simulink model "MotorControl"  (R2016a)
settings: Solver=VariableStepAuto  StartTime=0.0  StopTime=2  MaxStep=.01  RelTol=1e-3
libraries: simulink x3
settings Model: Creator=Dillon  LastModifiedBy=Dillon

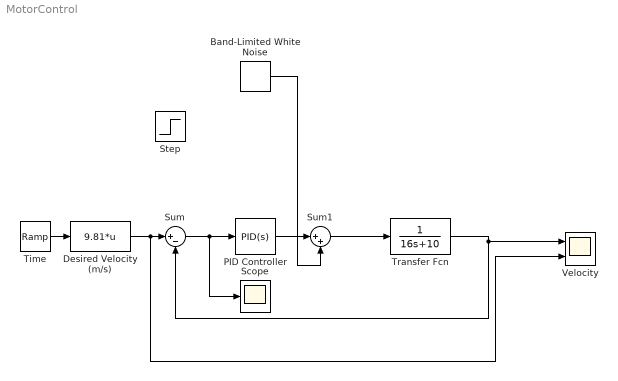
== system MotorControl ==
  Band-Limited White Noise : simulink/Sources/Band-Limited White Noise  Cov=[100]  Ts=0.1  seed=[23341]
  Desired Velocity (m/s) : Fcn  Expr=9.81*u
  PID Controller : simulink/Continuous/PID Controller  Controller=PID  TimeDomain=Continuous-time  SampleTime=-1  IntegratorMethod=Forward Euler  FilterMethod=Forward Euler  Form=Parallel  UseFilter=on  ControllerParametersSource=internal  P=100  I=1000  D=10  N=100  InitialConditionSource=internal  InitialConditionForIntegrator=0  InitialConditionForFilter=0  ExternalReset=none  LimitOutput=off  UpperSaturationLimit=inf  LowerSaturationLimit=-inf  LinearizeAsGain=on  AntiWindupMode=none  Kb=1  TrackingMode=off  Kt=1  PParamMin=[]  PParamMax=[]  IParamMin=[]  IParamMax=[]  DParamMin=[]  DParamMax=[]  NParamMin=[]  NParamMax=[]  KbParamMin=[]  KbParamMax=[]  KtParamMin=[]  KtParamMax=[]  POutMin=[]  POutMax=[]  IOutMin=[]  IOutMax=[]  DOutMin=[]  DOutMax=[]  NOutMin=[]  NOutMax=[]  KbOutMin=[]  KbOutMax=[]  KtOutMin=[]  KtOutMax=[]  IntegratorOutMin=[]  IntegratorOutMax=[]  FilterOutMin=[]  FilterOutMax=[]  SumOutMin=[]  SumOutMax=[]  SumI1OutMin=[]  SumI1OutMax=[]  SumI2OutMin=[]  SumI2OutMax=[]  SumI3OutMin=[]  SumI3OutMax=[]  SumDOutMin=[]  SumDOutMax=[]  SaturationOutMin=[]  SaturationOutMax=[]  IntegratorContinuousStateAttributes=''  IntegratorStateMustResolveToSignalObject=off  IntegratorRTWStateStorageClass=Auto  FilterContinuousStateAttributes=''  FilterStateMustResolveToSignalObject=off  FilterRTWStateStorageClass=Auto  DifferentiatorICPrevScaledInput=0  DifferentiatorOutMin=[]  DifferentiatorOutMax=[]
  Scope : Scope
  Step : Step  After=100  SampleTime=0
  Sum : Sum  Inputs=|+-
  Sum1 : Sum  Inputs=|++
  Time : simulink/Sources/Ramp  slope=1  start=0  X0=0
  Transfer Fcn : TransferFcn  Denominator=[16 10]
  Velocity : Scope  NumInputPorts=2
  wires:
  Time/1 -> Desired Velocity (m/s)/1
  Desired Velocity (m/s)/1 -> Velocity/2, Sum/1
  Sum/1 -> Scope/1, PID Controller/1
  Transfer Fcn/1 -> Sum/2, Velocity/1
  Sum1/1 -> Transfer Fcn/1
  PID Controller/1 -> Sum1/1
  Band-Limited White Noise/1 -> Sum1/2
